simulink model "sim_PIDHub"  (R2016b)
settings: Solver=VariableStepAuto  StartTime=0.0  StopTime=30.0  RelTol=1e-3
values from neighbouring files (symbols this model uses):
  matR_hub = 10000    [calcKalmanHub.m]
undefined symbols (not defined in the file or in its folder): Continuous, matA_hub_g, matB_hub, matB_hub_g, matC_hub_g, matE_hub, systemhub, Time
libraries: simulink x3, ctrlSharedLib x1
settings Model: Creator=nicol  LastModifiedBy=nicol

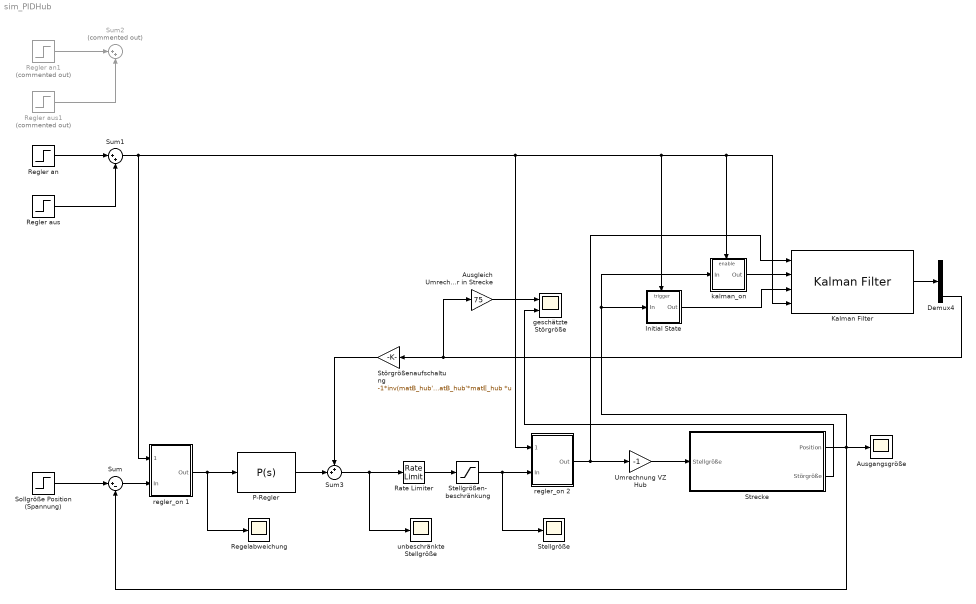
== system sim_PIDHub ==
  Ausgangsgröße : Scope
  Ausgleich Umrechnungsfaktor in Strecke : Gain  Gain=75
  Demux4 : Demux  Outputs=3
  Initial State : Subsystem  TreatAsAtomicUnit=on
  Kalman Filter : ctrlSharedLib/Kalman Filter  TimeDomain=Continuous-Time  UseCurrentEstimator=on  ModelSource=Individual A, B, C, D matrices  ModelSourceVariable=ss(0.95,1,1,0,1)  A=matA_hub_g  B=matB_hub_g  C=matC_hub_g  D=0  NumberOfStates=1  NumberOfInputs=1  NumberOfOutputs=1  InitialEstimateSource=Input port  X0=0  P0=10  UseK=off  UseGH=on  NumberOfProcessNoiseInputs=1  G=matG_hub  TimeInvariantG=on  H=0  TimeInvariantH=on  Q=matQ_hub  TimeInvariantQ=on  R=matR_hub  TimeInvariantR=on  N=0  TimeInvariantN=on  AddInputPort=on  AddEnablePort=off  ExternalReset=rising  OutputEstimatedY=off  OutputP=off  Ts=-1
  P-Regler : simulink/Continuous/PID Controller  Controller=P  TimeDomain=Continuous-time  SampleTime=-1  IntegratorMethod=Forward Euler  FilterMethod=Forward Euler  Form=Parallel  UseFilter=on  ControllerParametersSource=internal  P=0.8  I=0  D=0.1  N=100  InitialConditionSource=internal  InitialConditionForIntegrator=0  InitialConditionForFilter=0  ExternalReset=falling  LimitOutput=off  UpperSaturationLimit=inf  LowerSaturationLimit=-inf  LinearizeAsGain=on  AntiWindupMode=none  Kb=1  TrackingMode=on  Kt=2  PParamMin=[]  PParamMax=[]  IParamMin=[]  IParamMax=[]  DParamMin=[]  DParamMax=[]  NParamMin=[]  NParamMax=[]  KbParamMin=[]  KbParamMax=[]  KtParamMin=[]  KtParamMax=[]  POutMin=[]  POutMax=[]  IOutMin=[]  IOutMax=[]  DOutMin=[]  DOutMax=[]  NOutMin=[]  NOutMax=[]  KbOutMin=[]  KbOutMax=[]  KtOutMin=[]  KtOutMax=[]  IntegratorOutMin=[]  IntegratorOutMax=[]  FilterOutMin=[]  FilterOutMax=[]  SumOutMin=[]  SumOutMax=[]  SumI1OutMin=[]  SumI1OutMax=[]  SumI2OutMin=[]  SumI2OutMax=[]  SumI3OutMin=[]  SumI3OutMax=[]  SumDOutMin=[]  SumDOutMax=[]  SaturationOutMin=[]  SaturationOutMax=[]  IntegratorContinuousStateAttributes=''  IntegratorStateMustResolveToSignalObject=off  IntegratorRTWStateStorageClass=Auto  FilterContinuousStateAttributes=''  FilterStateMustResolveToSignalObject=off  FilterRTWStateStorageClass=Auto  DifferentiatorICPrevScaledInput=0  DifferentiatorOutMin=[]  DifferentiatorOutMax=[]
  Rate Limiter : RateLimiter  RisingSlewLimit=0.23024  FallingSlewLimit=-0.23024  SampleTimeMode=inherited
  Regelabweichung : Scope
  Regler an : Step  Time=0  SampleTime=0
  Regler an1 : Step  Commented=on  Time=16  SampleTime=0
  Regler aus : Step  Time=30  After=-1  SampleTime=0
  Regler aus1 : Step  Commented=on  Time=25  After=-1  SampleTime=0
  Sollgröße Position (Spannung) : Step  After=0.5  SampleTime=0
  Stellgröße : Scope
  Stellgrößen- beschränkung : Saturate  UpperLimit=1  LowerLimit=-1
  Strecke : Subsystem
  Störgrößenaufschaltung : Gain  Gain=-1*inv(matB_hub'*matB_hub)*matB_hub'*matE_hub  Multiplication=Matrix(K*u)
  Sum : Sum  Inputs=|+-
  Sum1 : Sum  Inputs=|++
  Sum2 : Sum  Commented=on  Inputs=|++
  Sum3 : Sum  Inputs=++|
  Umrechnung VZ Hub : Gain  Gain=-1
  geschätzte Störgröße : Scope  NumInputPorts=2
  kalman_on : Subsystem  TreatAsAtomicUnit=on
  regler_on 1 : Subsystem
  regler_on 2 : Subsystem
  unbeschränkte Stellgröße : Scope
  wires:
  Rate Limiter/1 -> Stellgrößen- beschränkung/1
  Stellgrößen- beschränkung/1 -> regler_on 2/2(In), Stellgröße/1
  Sollgröße Position (Spannung)/1 -> Sum/1
  Strecke/1(Position) -> Ausgangsgröße/1, Sum/2, Initial State/1(In), kalman_on/1(In)
  regler_on 2/1(Out) -> Kalman Filter/1, Umrechnung VZ Hub/1
  regler_on 1/1(Out) -> Regelabweichung/1, P-Regler/1
  Sum/1 -> regler_on 1/2(In)
  Regler an/1 -> Sum1/1
  Regler aus/1 -> Sum1/2
  Sum1/1 -> Initial State/Trigger, kalman_on/Enable, Kalman Filter/4, regler_on 2/1(regler_ on), regler_on 1/1(regler_ on)
  Regler an1/1 -> Sum2/1
  Regler aus1/1 -> Sum2/2
  P-Regler/1 -> Sum3/2
  Sum3/1 -> Rate Limiter/1, unbeschränkte Stellgröße/1
  Kalman Filter/1 -> Demux4/1
  Demux4/3 -> Ausgleich Umrechnungsfaktor in Strecke/1, Störgrößenaufschaltung/1
  kalman_on/1(Out) -> Kalman Filter/2
  Initial State/1(Out) -> Kalman Filter/3
  Strecke/2(Störgröße) -> geschätzte Störgröße/2
  Ausgleich Umrechnungsfaktor in Strecke/1 -> geschätzte Störgröße/1
  Umrechnung VZ Hub/1 -> Strecke/1(Stellgröße)
  Störgrößenaufschaltung/1 -> Sum3/1

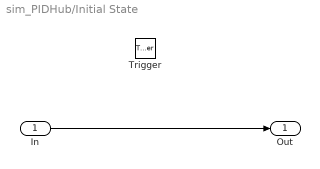
== system sim_PIDHub/Initial State ==
  In : Inport
  Trigger : TriggerPort  VariantControl=Variant
  Out : Outport
  wires:
  In/1 -> Out/1

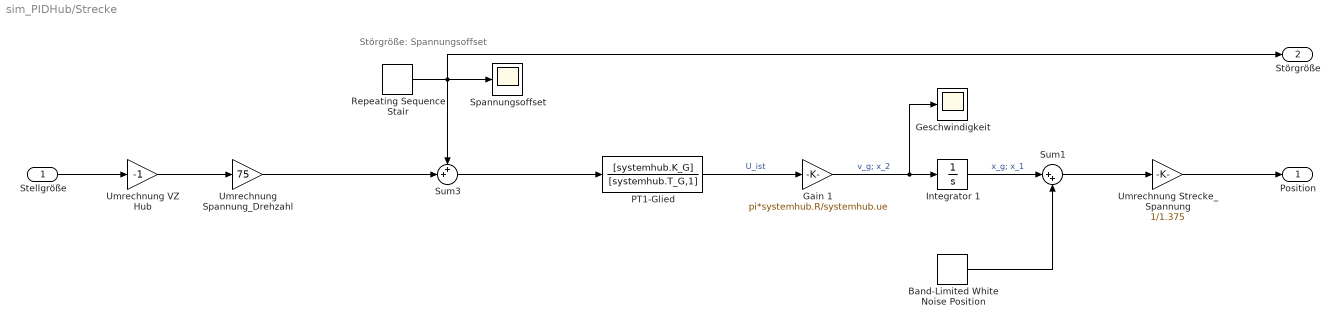
== system sim_PIDHub/Strecke ==
  note: Störgröße: Spannungsoffset
  Stellgröße : Inport
  Band-Limited White Noise Position : simulink/Sources/Band-Limited White Noise  Cov=[0.0000001]  Ts=0.01  seed=[23341]
  Gain 1 : Gain  Gain=pi*systemhub.R/systemhub.ue
  Geschwindigkeit : Scope
  Integrator 1 : Integrator
  PT1-Glied : TransferFcn  Numerator=[systemhub.K_G]  Denominator=[systemhub.T_G,1]
  Repeating Sequence Stair : simulink/Sources/Repeating Sequence Stair  OutValues=[0.02 0.05 0.05 0.02 0.08].'  tsamp=5  OutMin=[]  OutMax=[]  OutDataTypeStr=double  OutputDataTypeScalingMode=double  OutDataType=fixdt(0,8)  ConRadixGroup=Best Precision: Vector-wise  OutScaling=2^-12
  Spannungsoffset : Scope
  Sum1 : Sum  Inputs=|++
  Sum3 : Sum  Inputs=++|
  Umrechnung Spannung_Drehzahl : Gain  Gain=75
  Umrechnung Strecke_Spannung : Gain  Gain=1/1.375
  Umrechnung VZ Hub : Gain  Gain=-1
  Position : Outport
  Störgröße : Outport  Port=2
  wires:
  Sum3/1 -> PT1-Glied/1
  PT1-Glied/1 -> Gain 1/1  "U_ist"
  Gain 1/1 -> Geschwindigkeit/1, Integrator 1/1  "v_g; x_2"
  Integrator 1/1 -> Sum1/1  "x_g; x_1"
  Repeating Sequence Stair/1 -> Sum3/1, Störgröße/1, Spannungsoffset/1
  Umrechnung Spannung_Drehzahl/1 -> Sum3/2
  Sum1/1 -> Umrechnung Strecke_Spannung/1
  Band-Limited White Noise Position/1 -> Sum1/2
  Umrechnung Strecke_Spannung/1 -> Position/1
  Umrechnung VZ Hub/1 -> Umrechnung Spannung_Drehzahl/1
  Stellgröße/1 -> Umrechnung VZ Hub/1

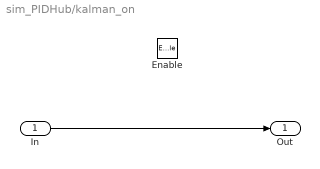
== system sim_PIDHub/kalman_on ==
  In : Inport
  Enable : EnablePort
  Out : Outport
  wires:
  In/1 -> Out/1

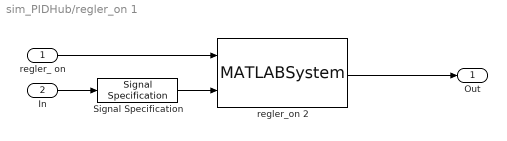
== system sim_PIDHub/regler_on 1 ==
  regler_ on : Inport
  In : Inport  Port=2
  Signal Specification : SignalSpecification  Dimensions=1
  regler_on 2 : MATLABSystem  System=regler_switch_1  SimulateUsing=Code generation
      mask Type: regler_switch_1
      mask Display:
      | disp('regler_switch_1');
      | port_label('input',1,'regler_on');
      | port_label('input',2,'input');
      | port_label('output',1,'y');
  Out : Outport
  wires:
  regler_ on/1 -> regler_on 2/1
  regler_on 2/1 -> Out/1
  Signal Specification/1 -> regler_on 2/2
  In/1 -> Signal Specification/1

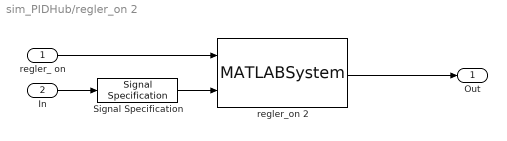
== system sim_PIDHub/regler_on 2 ==
  regler_ on : Inport
  In : Inport  Port=2
  Signal Specification : SignalSpecification  Dimensions=1
  regler_on 2 : MATLABSystem  System=regler_switch_1  SimulateUsing=Code generation
      mask Type: regler_switch_1
      mask Display:
      | disp('regler_switch_1');
      | port_label('input',1,'regler_on');
      | port_label('input',2,'input');
      | port_label('output',1,'y');
  Out : Outport
  wires:
  regler_ on/1 -> regler_on 2/1
  regler_on 2/1 -> Out/1
  Signal Specification/1 -> regler_on 2/2
  In/1 -> Signal Specification/1
